simulink model "s_ident4"  (Simulink 4.00)
settings: Solver=ode45  StartTime=0.0  StopTime=100  RelTol=1e-3
libraries: slident x1
settings Model: LastModifiedBy=Administrator  BlockReductionOpt=off

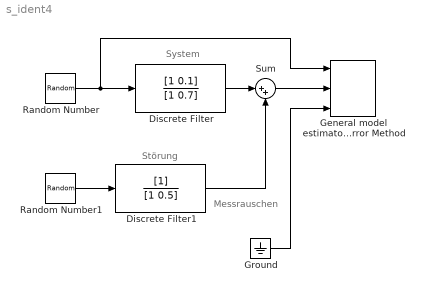
== system s_ident4 ==
  note: Messrauschen
  note: System
  note: Störung
  Discrete Filter : DiscreteFilter  Numerator=[1 0.1]  Denominator=[1 0.7]  SampleTime=0.1  Realization=auto
  Discrete Filter1 : DiscreteFilter  Numerator=[1]  Denominator=[1 0.5]  SampleTime=0.1  Realization=auto
  General model estimator using Predictive Error Method : slident/General model estimator using Predictive Error Method  MaskParam1=256  MaskParam2=[1 2 0 0 0 0]  MaskParam3=64  MaskParam4=0.1
  Ground : Ground
  Random Number : RandomNumber  Mean=0  Variance=1  Seed=0  SampleTime=0.1
  Random Number1 : RandomNumber  Mean=0  Variance=1  Seed=1479  SampleTime=0.1
  Sum : Sum  Inputs=|++  SaturateOnIntegerOverflow=on
  wires:
  Random Number/1 -> Discrete Filter/1, General model estimator using Predictive Error Method/1
  Random Number1/1 -> Discrete Filter1/1
  Discrete Filter/1 -> Sum/1
  Sum/1 -> General model estimator using Predictive Error Method/2
  Discrete Filter1/1 -> Sum/2
  Ground/1 -> General model estimator using Predictive Error Method/3
